simulink library "mylib"  (R2021a)
settings: Solver=VariableStepAuto  StartTime=0.0  StopTime=10.0  RelTol=1e-3
settings Model: Creator=prasad  LastModifiedBy=prasad

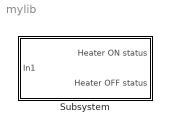
== system mylib ==
  Subsystem : Subsystem

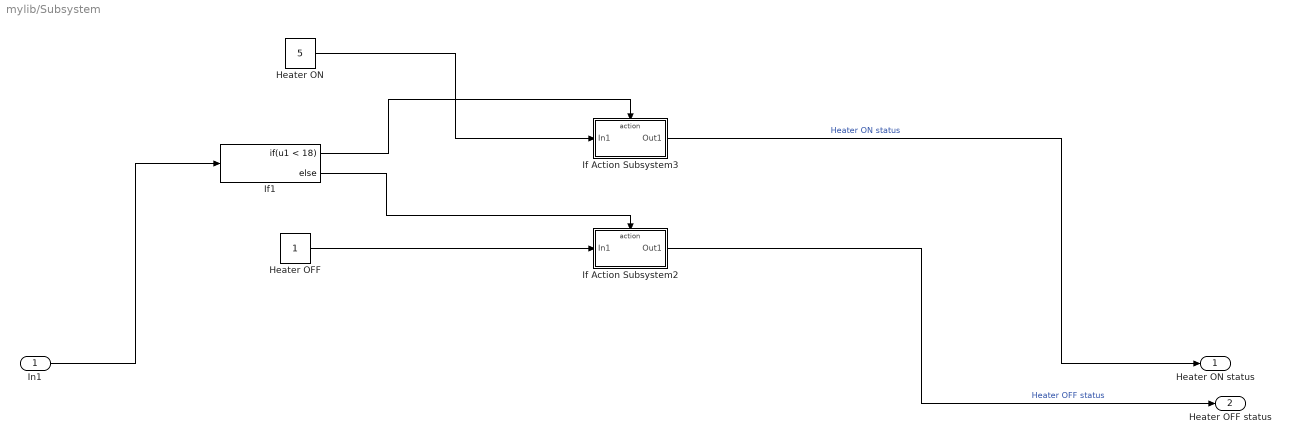
== system mylib/Subsystem ==
  In1 : Inport
  Heater OFF : Constant
  Heater ON : Constant  Value=5
  If Action Subsystem2 : Subsystem  TreatAsAtomicUnit=on
  If Action Subsystem3 : Subsystem  TreatAsAtomicUnit=on
  If1 : If  IfExpression=u1 < 18
  Heater ON status : Outport
  Heater OFF status : Outport  Port=2
  wires:
  In1/1 -> If1/1
  If1/1 -> If Action Subsystem3/Action
  Heater OFF/1 -> If Action Subsystem2/1(In1)
  Heater ON/1 -> If Action Subsystem3/1(In1)
  If Action Subsystem2/1(Out1) -> Heater OFF status/1  "Heater OFF status"
  If Action Subsystem3/1(Out1) -> Heater ON status/1  "Heater ON status"
  If1/2 -> If Action Subsystem2/Action

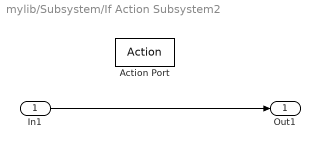
== system mylib/Subsystem/If Action Subsystem2 ==
  In1 : Inport
  Action Port : ActionPort  ActionPortLabel=else
  Out1 : Outport
  wires:
  In1/1 -> Out1/1

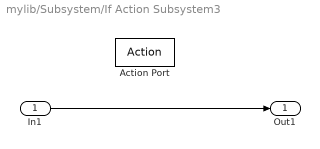
== system mylib/Subsystem/If Action Subsystem3 ==
  In1 : Inport
  Action Port : ActionPort  ActionPortLabel=if(u1 < 18)
  Out1 : Outport
  wires:
  In1/1 -> Out1/1
